simulink model "test12_1"  (R2024a)
settings: Solver=FixedStepAuto  StartTime=0.0  StopTime=30  FixedStep=0.001  MaxStep=1e-2  RelTol=1e-3
libraries: fl_lib x21, nesl_utility x14, sdl_lib x8, simulink x4
(part 2 of 2)

== matlab function test12_1/Clutch/MATLAB Function2 ==
  data: boundary input; output_torque output; input_torque input
function output_torque = fcn(boundary, input_torque)

if boundary <= 0
    output_torque = 0;
else
    if abs(input_torque) <= boundary
        output_torque = input_torque;
    else
        if input_torque > 0
           output_torque = boundary;
        else
        output_torque = -1 * boundary;
        end
    end
end

== matlab function test12_1/Clutch/MATLAB Function ==
  data: Gear_1 input; Gear_Shifting output; Gear_2 input; Speed input
function Gear_Shifting = fcn(Gear_1, Gear_2, Speed)

if (Gear_2 > 4500)||(Speed > 60)
    Gear_Shifting = 2;
else
    Gear_Shifting = 1;
end

== matlab function test12_1/Gear Shifting Strategy/MATLAB Function ==
  data: Gear_Shift input; Integrator input; Output_Current output
function Output_Current  = fcn(Gear_Shift, Integrator)

if Gear_Shift == 1
    Output_Current = 10;
else
    Output_Current = Integrator;
end

== matlab function test12_1/Subsystem/MATLAB Function3 ==
  data: u input; y output
function y = fcn(u)

if u < -200
    y = -200;
elseif u> 200
    y = 200;
else
    y = u;
end

== matlab function test12_1/MATLAB Function ==
  data: Gear_Shift input; Clutch_One_Current output; Shift_One_Current input; Shift_Two_Current input; Clutch_Two_Current output; Stable output
function [Clutch_One_Current, Clutch_Two_Current, Stable] = fcn(Gear_Shift, Shift_One_Current, Shift_Two_Current)

if Gear_Shift == 1
    if Shift_Two_Current > 1
            Clutch_Two_Current = 1;
            Clutch_One_Current = 2;
            Stable = 1;
    else
             Clutch_Two_Current = 0;
             Clutch_One_Current = 2;
             Stable = 0;
    end
else
    if Shift_One_Current > 1
            Clutch_One_Current = 1;
            Clutch_Two_Current = 2;
            Stable = 1;
    else
             Clutch_One_Current = 0;
             Clutch_Two_Current = 2;
             Stable = 0;
    end
end

== matlab function test12_1/MATLAB Function1 ==
  data: Stable input; Output output; Torque input; Last_Torque input
function Output = fcn(Stable, Torque, Last_Torque)

if Stable == 1
    Output = Torque;
else
    Output = Last_Torque;
end

== matlab function test12_1/MATLAB Function2 ==
  data: Free_Shift input; Shift_One output; Contral_Shift input; Gear_Shift input; Shift_Two output
function [Shift_One, Shift_Two] = fcn(Free_Shift, Contral_Shift, Gear_Shift)

if Gear_Shift == 1
    Shift_One = Contral_Shift;
    Shift_Two = Free_Shift;
else
    Shift_One = Free_Shift;
    Shift_Two = Contral_Shift;
end

== matlab function test12_1/MATLAB Function3 ==
  data: a input; y output; b input; Stable input
function y = fcn(a,b,Stable)

if Stable == 1
    y = a;
else
    y = b;
end
